simulink library "MyLibNova"  (R2024b)
settings: Solver=VariableStepAuto  StartTime=0.0  StopTime=10.0  RelTol=1e-3
settings Model: Creator=chall  LastModifiedBy=chall

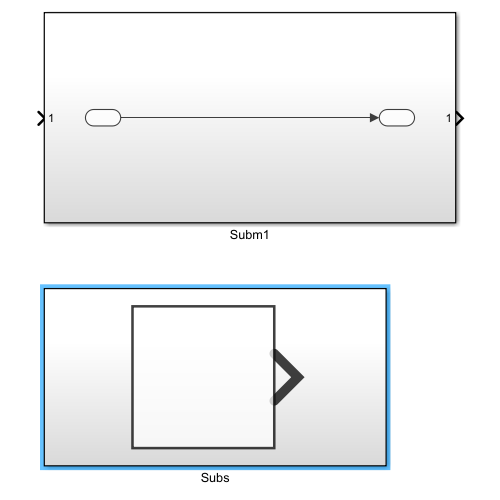
[thumbnail: Simulink's stored preview of the top-level diagram]
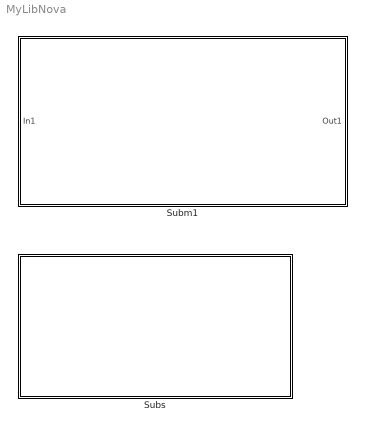
== system MyLibNova ==
  Subm1 : Subsystem
  Subs : Subsystem

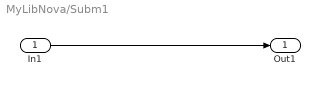
== system MyLibNova/Subm1 ==
  In1 : Inport
  Out1 : Outport
  wires:
  In1/1 -> Out1/1

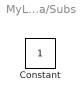
== system MyLibNova/Subs ==
  Constant : Constant
